simulink model "fcn-DESKTOP-1TKS2SV"  (R2021a)
settings: Solver=VariableStepAuto  StartTime=0.0  StopTime=27  MaxStep=0.54  RelTol=1e-3
values from neighbouring files (symbols this model uses):
  Ar = pi*R_rad^2    (= 0.00282743338823)    [constants1DoF.m]
  Cd = 0.5    [constants1DoF.m]
  g = 9.81    [constants1DoF.m]
  m_d_c = 0.01    [constants1DoF.m]
  m_r = 0.5    [constants1DoF.m]
  rho = 1.225    [constants1DoF.m]
  t_burn = 2    [constants1DoF.m]
  Tmax = 10    [constants1DoF.m]
settings Model: Creator=josepfamador  LastModifiedBy=josep
settings SolverCC: AlgebraicLoopSolver=TrustRegion
settings DebuggingCC: SFMachineParentedDataDiag=warning

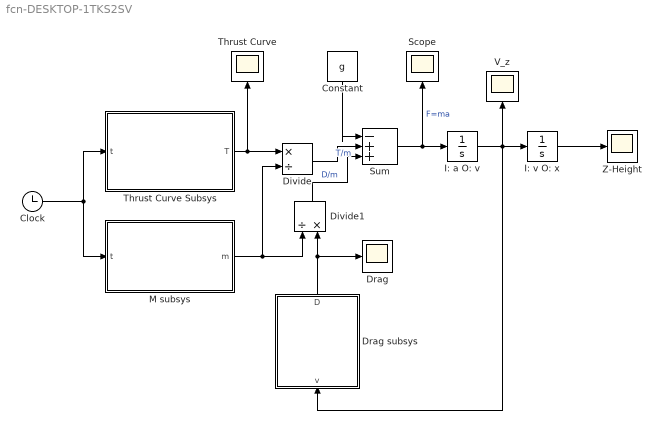
== system fcn-DESKTOP-1TKS2SV ==
  Clock : Clock
      settings: Decimation=5
  Constant : Constant  Value=g
  Divide : Product  Inputs=*/
  Divide1 : Product  Inputs=/*
  Drag : Scope
  Drag subsys : Subsystem
  I: a O: v : Integrator
  I: v O: x : Integrator
  M subsys : Subsystem
  Scope : Scope
  Sum : Sum  Inputs=|-++
  Thrust Curve : Scope
  Thrust Curve Subsys : Subsystem
  V_z : Scope
  Z-Height : Scope
  wires:
  Clock/1 -> Thrust Curve Subsys/1(t), M subsys/1(t)
  Constant/1 -> Sum/1
  Sum/1 -> I: a O: v/1, Scope/1  "F=ma"
  I: v O: x/1 -> Z-Height/1
  I: a O: v/1 -> Drag subsys/1(v), V_z/1, I: v O: x/1
  Divide/1 -> Sum/2  "T/m"
  Divide1/1 -> Sum/3  "D/m"
  M subsys/1(m) -> Divide1/1, Divide/2
  Thrust Curve Subsys/1(T) -> Thrust Curve/1, Divide/1
  Drag subsys/1(D) -> Drag/1, Divide1/2

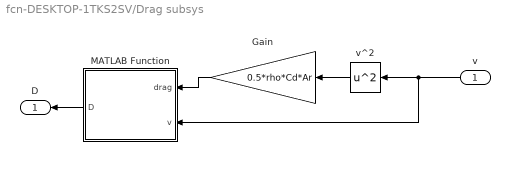
== system fcn-DESKTOP-1TKS2SV/Drag subsys ==
  v : Inport
  Gain : Gain  Gain=0.5*rho*Cd*Ar
  MATLAB Function : MATLAB Function  TreatAsAtomicUnit=on
  v^2 : Math  Operator=square  SaturateOnIntegerOverflow=on
  D : Outport
  wires:
  v^2/1 -> Gain/1
  v/1 -> MATLAB Function/2(v), v^2/1
  Gain/1 -> MATLAB Function/1(drag)
  MATLAB Function/1(D) -> D/1

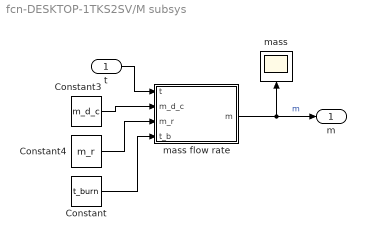
== system fcn-DESKTOP-1TKS2SV/M subsys ==
  t : Inport
  Constant : Constant  Value=t_burn
  Constant3 : Constant  Value=m_d_c
  Constant4 : Constant  Value=m_r
  mass : Scope
  mass flow rate : MATLAB Function  TreatAsAtomicUnit=on
  m : Outport
  wires:
  t/1 -> mass flow rate/1(t)
  Constant3/1 -> mass flow rate/2(m_d_c)
  Constant4/1 -> mass flow rate/3(m_r)
  mass flow rate/1(m) -> m/1, mass/1  "m"
  Constant/1 -> mass flow rate/4(t_b)

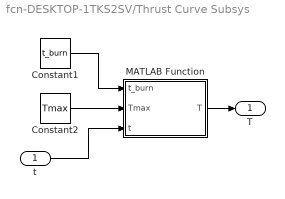
== system fcn-DESKTOP-1TKS2SV/Thrust Curve Subsys ==
  t : Inport
  Constant1 : Constant  Value=t_burn
  Constant2 : Constant  Value=Tmax
  MATLAB Function : MATLAB Function  TreatAsAtomicUnit=on
  T : Outport
  wires:
  Constant1/1 -> MATLAB Function/1(t_burn)
  Constant2/1 -> MATLAB Function/2(Tmax)
  t/1 -> MATLAB Function/3(t)
  MATLAB Function/1(T) -> T/1

== matlab function fcn-DESKTOP-1TKS2SV/M subsys/mass flow rate ==
  data: t input; m output; m_d_c input; m_r input; t_b input
function m = m_flow(t, m_d_c, m_r, t_b)
%Const Define in 'constants1DoF.m'
%out mass at time t


if t <= t_b 
    m= -m_d_c*t + m_r;
else
    m = -m_d_c*t_b + m_r;
end

== matlab function fcn-DESKTOP-1TKS2SV/Thrust Curve Subsys/MATLAB Function ==
  data: t_burn input; Tmax input; t input; T output
function T = T_of_t(t_burn, Tmax, t)
%Approx Thurst Curve.
%Total Burn time = 1s
%Max Thrust 100N
%Constants Defined in 'constants1DoF.m'
x_hf = t_burn/2;
a = Tmax/((x_hf)*(x_hf - t_burn));


if t<=0 || t>t_burn
    T = 0;
else
    T = a*t*(t-t_burn);
end

== matlab function fcn-DESKTOP-1TKS2SV/Drag subsys/MATLAB Function ==
  data: drag input; D output; v input
function D = sign_change(drag, v)
%changes signs of Drag when appropiate. Vertical Up is positive
if v>0
    D = -drag;
else
    D = drag;
end
